simulink model "bicyclemodel"  (R2026a)
settings: Solver=VariableStepAuto
settings Model: Creator=eonra  LastModifiedBy=eonra

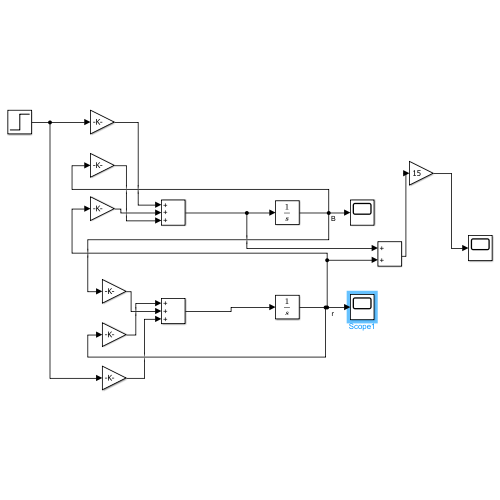
[thumbnail: Simulink's stored preview of the top-level diagram]
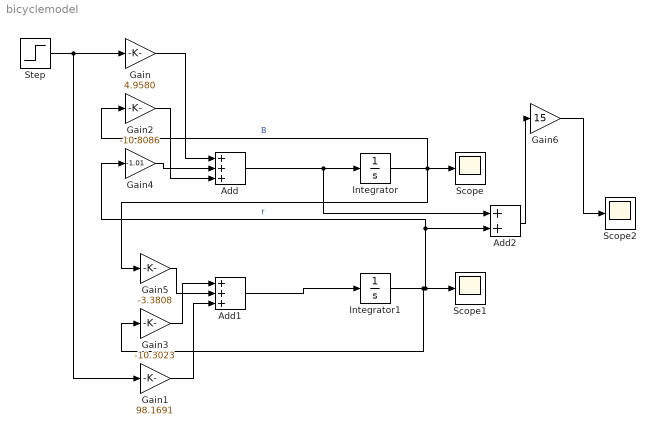
== system bicyclemodel ==
  Add : Sum  Inputs=+++
  Add1 : Sum  Inputs=+++
  Add2 : Sum
  Gain : Gain  Gain=4.9580
  Gain1 : Gain  Gain=98.1691
  Gain2 : Gain  Gain=-10.8086
  Gain3 : Gain  Gain=-10.3023
  Gain4 : Gain  Gain=-1.01
  Gain5 : Gain  Gain=-3.3808
  Gain6 : Gain  Gain=15
  Integrator : Integrator
  Integrator1 : Integrator
  Scope : Scope
      settings: ActiveDisplayYMinimum=-0.04399720841288509  ActiveDisplayYMaximum=0.014368420530596658
  Scope1 : Scope
      settings: ActiveDisplayYMinimum=-0.0982012810679967  ActiveDisplayYMaximum=0.88381152961197063
  Scope2 : Scope
      settings: ActiveDisplayYMinimum=-1.4730192160241924  ActiveDisplayYMaximum=13.257172944217734  DataLoggingVariableName=ScopeData2
  Step : Step  FinalValue=0.0812  SampleTime=0
  wires:
  Integrator/1 -> Gain5/1, Gain2/1, Scope/1  "B"
  Integrator1/1 -> Gain3/1, Add2/2, Gain4/1, Scope1/1  "r"
  Step/1 -> Gain1/1, Gain/1
  Gain1/1 -> Add1/3
  Gain/1 -> Add/1
  Add/1 -> Add2/1, Integrator/1
  Add1/1 -> Integrator1/1
  Gain3/1 -> Add1/1
  Gain2/1 -> Add/3
  Gain5/1 -> Add1/2
  Gain4/1 -> Add/2
  Add2/1 -> Gain6/1
  Gain6/1 -> Scope2/1
